simulink model "rocketLIBRARY"  (R2023a)
settings: Solver=VariableStepAuto  StartTime=0.0  StopTime=70  RelTol=1e-3
undefined symbols (not defined in the file or in its folder): Earth, magnitude, WGS84
libraries: aerolibanim x1, aerolibadyn x1, aerolibtransform2 x1, aerolibfltsims x1, aerolibatmos2 x1, shared6dof x1, aerolibwind2 x1
settings Model: Creator=User  LastModifiedBy=User

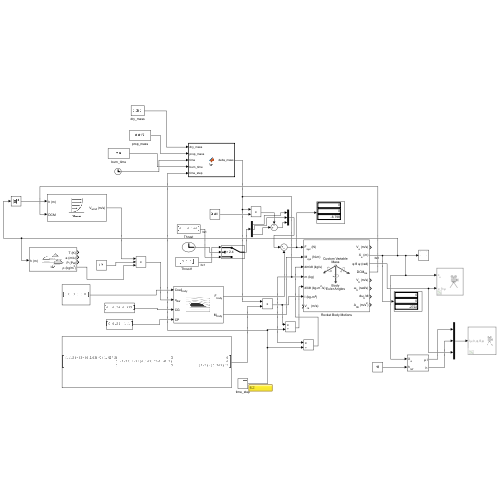
[thumbnail: Simulink's stored preview of the top-level diagram]
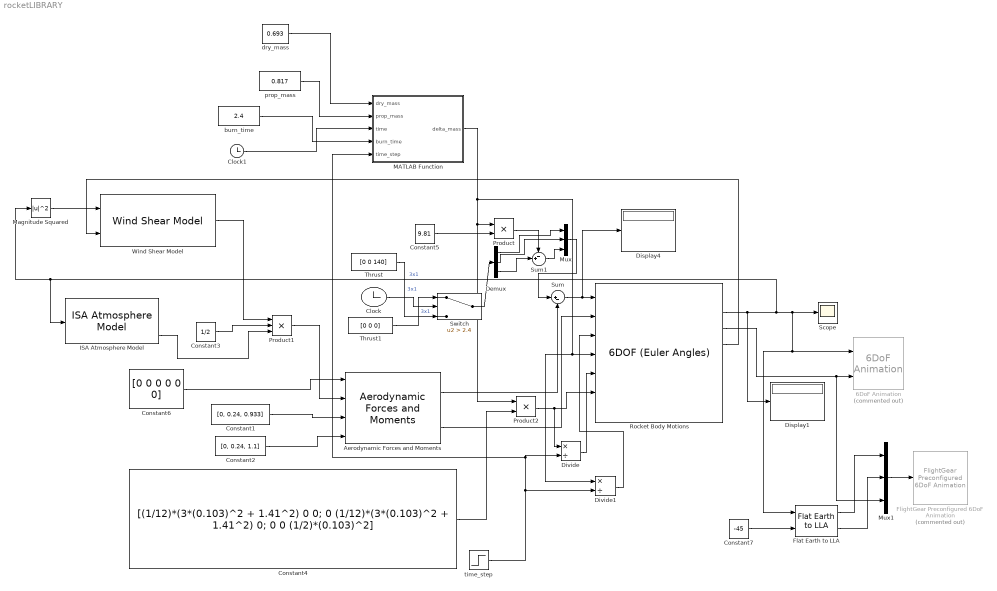
== system rocketLIBRARY ==
  6DoF Animation : aerolibanim/6DoF Animation  Commented=on  u1=[-1000 1000 -500 500 0 3000]  u2=0.1  u3=1.0  u4=[4000 0 -5000]  u5=Fixed position  u6=[2000 500 -3150]  u7=10  u8=on
  "Aerodynamic Forces and Moments " : aerolibadyn/Aerodynamic Forces and Moments   inputAxes=Body  outputForceAxes=Body  outputMomentAxes=Body  S=pi*(24/100)^2  b=0  cbar=0
  Clock : Clock
  Clock1 : Clock
  Constant1 : Constant  Value=[0, 0.24, 0.933]
  Constant2 : Constant  Value=[0, 0.24, 1.1]
  Constant3 : Constant  Value=1/2
  Constant4 : Constant  Value=[(1/12)*(3*(0.103)^2 + 1.41^2) 0 0; 0 (1/12)*(3*(0.103)^2 + 1.41^2) 0; 0 0 (1/2)*(0.103)^2]
  Constant5 : Constant  Value=9.81
  Constant6 : Constant  Value=[0 0 0 0 0 0]
  Constant7 : Constant  Value=-45
  Demux : Demux  Outputs=3
  Display1 : Display
  Display4 : Display
  Divide : Product  Inputs=*/
  Divide1 : Product  Inputs=*/
  Flat Earth to LLA : aerolibtransform2/Flat Earth to LLA  units=Metric (MKS)  ptype=Earth (WGS84)  F=1/298.257223563  R=6378137  refPosPort=off  LL0=[0 10]  psi=0
  FlightGear Preconfigured 6DoF Animation : aerolibfltsims/FlightGear Preconfigured 6DoF Animation  Commented=on  xFlightGearVersion=v2019.1  DestinationIpAddress=127.0.0.1  DestinationPort=5502  SampleTime=1/30  packetVersion=24
  ISA Atmosphere Model : aerolibatmos2/ISA Atmosphere Model  custom=off  g=9.80665  gamma=1.4  R=287.0531  L=0.0065  h_trop=11000  h_strat=20000  rho0=1.225  P0=101325  T0=288.15  h0=0
  MATLAB Function : MATLAB Function  TreatAsAtomicUnit=on
  Magnitude Squared : Math  Operator=magnitude^2
  Mux : Mux  Inputs=3
  Mux1 : Mux  Inputs=3
  Product : Product
  Product1 : Product  Inputs=3
  Product2 : Product
  Rocket Body Motions : shared6dof/6DOF (Euler Angles)  units=Metric (MKS)  mtype=Custom Variable  rep=Euler Angles  xme_0=[0 0 0]  Vm_0=[0 0 0]  eul_0=[0 0 0]  pm_0=[0 0 0]  mass_0=1.517  mass_e=0.5  mass_f=2.0  inertia=eye(3)  inertia_e=eye(3)  inertia_f=2*eye(3)  k_quat=1.0  vre_flag=on  abi_flag=off  aMode=0  xme_statename=''  Vm_statename=''  eul_statename=''  quat_statename=''  pm_statename=''  mass_statename=''
  Scope : Scope
  Sum : Sum  Inputs=|+-
  Sum1 : Sum  Inputs=-+|
  Switch : Switch  Criteria=u2 > Threshold  Threshold=2.4  ZeroCross=off  SaturateOnIntegerOverflow=off  InputSameDT=off
  Thrust : Constant  Value=[0 0 140]
  Thrust1 : Constant  Value=[0 0 0]
  Wind Shear Model : aerolibwind2/Wind Shear Model  units=Metric (MKS)  phase=Category C - Terminal Flight Phase  W_20=15  Wdeg=0
  burn_time : Constant  Value=2.4
  dry_mass : Constant  Value=0.693
  prop_mass : Constant  Value=0.817
  time_step : Step  Time=0.01  Before=0.01  After=70  SampleTime=0
  wires:
  Rocket Body Motions/2 -> Magnitude Squared/1, ISA Atmosphere Model/1, Flat Earth to LLA/1, 6DoF Animation/1, Scope/1, Display1/1  "3x1"
  Sum/1 -> Display4/1, Rocket Body Motions/1
  Constant5/1 -> Product/2
  dry_mass/1 -> MATLAB Function/1(dry_mass)
  Product/1 -> Sum1/1
  Constant1/1 -> "Aerodynamic Forces and Moments "/3
  Constant2/1 -> "Aerodynamic Forces and Moments "/4
  Product1/1 -> "Aerodynamic Forces and Moments "/2
  Constant3/1 -> Product1/2
  ISA Atmosphere Model/4 -> Product1/3
  Constant4/1 -> Product2/2
  Product2/1 -> Divide/1, Rocket Body Motions/6
  "Aerodynamic Forces and Moments "/1 -> Sum/2
  Constant6/1 -> "Aerodynamic Forces and Moments "/1
  Rocket Body Motions/4 -> Wind Shear Model/2
  Wind Shear Model/1 -> Product1/1
  Magnitude Squared/1 -> Wind Shear Model/1
  Thrust1/1 -> Switch/1  "3x1"
  Switch/1 -> Demux/1
  Clock/1 -> Switch/2
  Rocket Body Motions/3 -> Mux1/3, 6DoF Animation/2
  Thrust/1 -> Switch/3  "3x1"
  Demux/2 -> Mux/2
  Demux/3 -> Sum1/2
  Sum1/1 -> Mux/3
  Demux/1 -> Mux/1
  Mux/1 -> Sum/1
  Flat Earth to LLA/2 -> Mux1/2
  Flat Earth to LLA/1 -> Mux1/1
  Mux1/1 -> FlightGear Preconfigured 6DoF Animation/1
  Constant7/1 -> Flat Earth to LLA/2
  prop_mass/1 -> MATLAB Function/2(prop_mass)
  burn_time/1 -> MATLAB Function/4(burn_time)
  Clock1/1 -> MATLAB Function/3(time)
  MATLAB Function/1(delta_mass) -> Rocket Body Motions/4, Divide1/1, Product/1, Product2/1
  time_step/1 -> MATLAB Function/5(time_step), Divide/2, Divide1/2
  Divide/1 -> Rocket Body Motions/5
  Divide1/1 -> Rocket Body Motions/3
  "Aerodynamic Forces and Moments "/2 -> Rocket Body Motions/2

== matlab function rocketLIBRARY/MATLAB Function ==
  data: dry_mass input; delta_mass output; prop_mass input; time input; burn_time input; time_step input
function delta_mass = fcn(dry_mass, prop_mass, time, burn_time, time_step)

mass = dry_mass; % Initial total mass of the rocket
prop_burn_rate = prop_mass / burn_time; % Propellant burn rate per unit time

% mass = initial_mass;

dt = time_step;

while time < burn_time
    prop_burned = prop_burn_rate * time; % Calculate the amount of propellant burned
    mass = mass + (prop_mass - prop_burned); % Update the total mass
    time = time + dt; % Increment time (assuming discrete time steps)
end


delta_mass = mass; % Calculate the change in mass
